simulink model "thermal_simulink_acados"  (R2017b)
settings: Solver=FixedStepDiscrete  StartTime=0.0  StopTime=500  FixedStep=1  RelTol=1e-3
values from neighbouring files (symbols this model uses):
  A_d = [0.386994154142 0.130528867937 0.00753731445977 1.05252849992e-06 0 0 0 0 0 0 0 -0.260915565234 ... (121 elements, 11x11)]    [battery_final_discrete_for_simulink.mat]    (also in convert_c2d.m = battery_sys_d.A)
  B_d = [0.00407902712304 0.000471082153736 1.68404559988e-05 1.71473651939e-09 0 0 0 0 0 0 0 0 ... (44 elements, 11x4)]    [battery_final_discrete_for_simulink.mat]    (also in convert_c2d.m = battery_sys_d.B)
  C_d = [-0.0403469184323 0 0.00489964923997 0 -0.00193385654799 0 0.0091411610057 0 0.0963442624262 0 0.00960199809146 0 ... (22 elements, 2x11)]    [battery_final_discrete_for_simulink.mat]    (also in convert_c2d.m = battery_sys_d.C)
  D_d = [0  0  0  0; 0  0  0  0]    [battery_final_discrete_for_simulink.mat]    (also in convert_c2d.m = battery_sys_d.D)
  nx_final = 11    [battery_final_portable_mux_demux_model.mat]
undefined symbols (not defined in the file or in its folder): DiscIntNeverNeededParam, disturbance_values
libraries: cstblocks x1, simulink x1
settings Model: Creator=dhruvkumar.patel  LastModifiedBy=dhruvkumar.patel

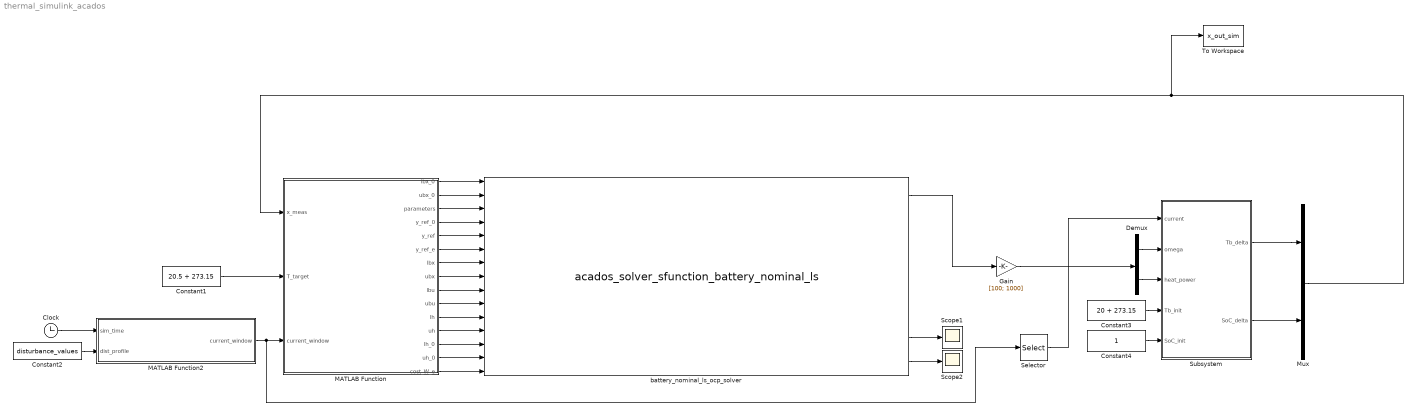
== system thermal_simulink_acados ==
  Clock : Clock
  Constant1 : Constant  Value=20.5 + 273.15
  Constant2 : Constant  Value=disturbance_values
  Constant3 : Constant  Value=20 + 273.15
  Constant4 : Constant
  Demux : Demux  Outputs=2
  Gain : Gain  Gain=[100; 1000]
  MATLAB Function : MATLAB Function  TreatAsAtomicUnit=on
  MATLAB Function2 : MATLAB Function  TreatAsAtomicUnit=on
  Mux : Mux  Inputs=2
  Scope1 : Scope
  Scope2 : Scope
  Selector : Selector  InputPortWidth=81  IndexOptions=Index vector (dialog)  Indices=1  OutputSizes=1
  Subsystem : Subsystem
  To Workspace : ToWorkspace  VariableName=x_out_sim  SampleTime=-1
  battery_nominal_ls_ocp_solver : S-Function  FunctionName=acados_solver_sfunction_battery_nominal_ls  SFunctionDeploymentMode=off  EnableBusSupport=off
      mask Display:
      | global sfun_input_names sfun_output_names
      | for i = 1:length(sfun_input_names)
      |     port_label('input', i, sfun_input_names{i})
      | end
      | for i = 1:length(sfun_output_names)
      |     port_label('output', i, sfun_output_names{i})
      | end
      | disp("acados OCP")
  wires:
  MATLAB Function/6(y_ref_e) -> battery_nominal_ls_ocp_solver/6
  MATLAB Function/5(y_ref) -> battery_nominal_ls_ocp_solver/5
  MATLAB Function/4(y_ref_0) -> battery_nominal_ls_ocp_solver/4
  MATLAB Function/3(parameters) -> battery_nominal_ls_ocp_solver/3
  MATLAB Function/2(ubx_0) -> battery_nominal_ls_ocp_solver/2
  MATLAB Function/1(lbx_0) -> battery_nominal_ls_ocp_solver/1
  MATLAB Function/7(lbx) -> battery_nominal_ls_ocp_solver/7
  MATLAB Function/8(ubx) -> battery_nominal_ls_ocp_solver/8
  MATLAB Function/9(lbu) -> battery_nominal_ls_ocp_solver/9
  MATLAB Function/10(ubu) -> battery_nominal_ls_ocp_solver/10
  MATLAB Function/11(lh) -> battery_nominal_ls_ocp_solver/11
  MATLAB Function/12(uh) -> battery_nominal_ls_ocp_solver/12
  MATLAB Function/13(lh_0) -> battery_nominal_ls_ocp_solver/13
  MATLAB Function/14(uh_0) -> battery_nominal_ls_ocp_solver/14
  MATLAB Function/15(cost_W_e) -> battery_nominal_ls_ocp_solver/15
  Constant1/1 -> MATLAB Function/2(T_target)
  MATLAB Function2/1(current_window) -> Selector/1, MATLAB Function/3(current_window)
  Clock/1 -> MATLAB Function2/1(sim_time)
  Constant2/1 -> MATLAB Function2/2(dist_profile)
  battery_nominal_ls_ocp_solver/7 -> Scope1/1
  battery_nominal_ls_ocp_solver/8 -> Scope2/1
  battery_nominal_ls_ocp_solver/1 -> Gain/1
  Gain/1 -> Demux/1
  Demux/1 -> Subsystem/2(omega)
  Demux/2 -> Subsystem/3(heat_power)
  Selector/1 -> Subsystem/1(current)
  Mux/1 -> To Workspace/1, MATLAB Function/1(x_meas)
  Subsystem/1(Tb_delta) -> Mux/1
  Subsystem/2(SoC_delta) -> Mux/2
  Constant3/1 -> Subsystem/4(Tb_init)
  Constant4/1 -> Subsystem/5(SoC_init)

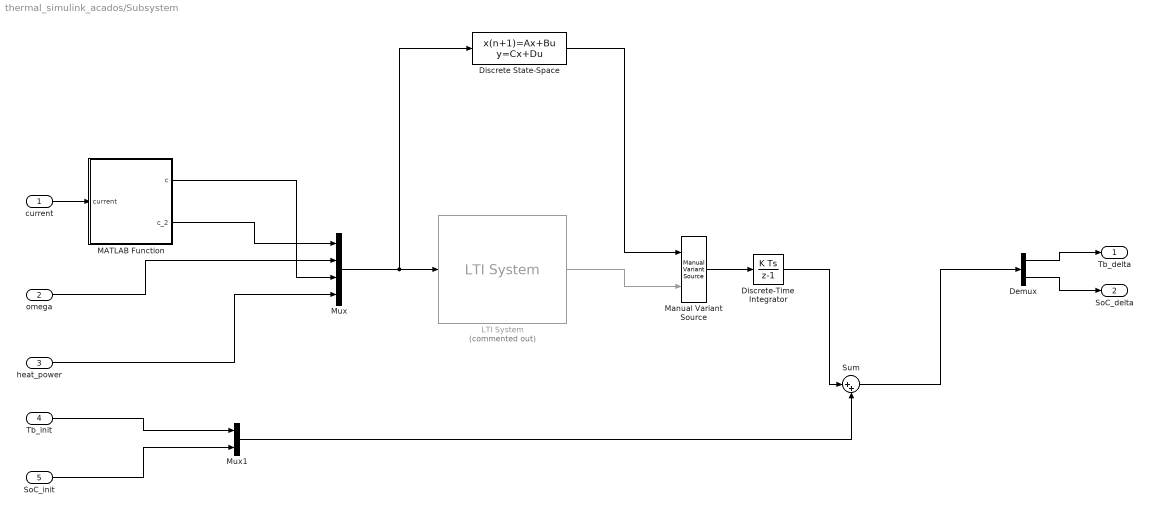
== system thermal_simulink_acados/Subsystem ==
  current : Inport
  omega : Inport  Port=2
  heat_power : Inport  Port=3
  Tb_init : Inport  Port=4
  SoC_init : Inport  Port=5
  Demux : Demux  Outputs=2
  Discrete State-Space : DiscreteStateSpace  A=A_d  B=B_d  C=C_d  D=D_d  InitialCondition=zeros(nx_final,1)  SampleTime=-1
  Discrete-Time Integrator : DiscreteIntegrator  InitialConditionSetting=State (most efficient)  SampleTime=-1  ICPrevOutput=DiscIntNeverNeededParam  ICPrevScaledInput=DiscIntNeverNeededParam
  LTI System : cstblocks/LTI System  Commented=on  sys=TF_final  IC=[]
  MATLAB Function : MATLAB Function  TreatAsAtomicUnit=on
  Manual Variant Source : simulink/Signal Routing/Manual Variant Source  NumChoices=2  OverrideUsingVariant=V_1
      settings: SourceProductName=Simulink
  Mux : Mux
  Mux1 : Mux  Inputs=2
  Sum : Sum  Inputs=|++
  Tb_delta : Outport
  SoC_delta : Outport  Port=2
  wires:
  current/1 -> MATLAB Function/1(current)
  Mux/1 -> Discrete State-Space/1, LTI System/1
  MATLAB Function/1(c) -> Mux/3
  Demux/2 -> SoC_delta/1
  Demux/1 -> Tb_delta/1
  MATLAB Function/2(c_2) -> Mux/1
  Manual Variant Source/1 -> Discrete-Time Integrator/1
  heat_power/1 -> Mux/4
  omega/1 -> Mux/2
  Discrete State-Space/1 -> Manual Variant Source/1
  LTI System/1 -> Manual Variant Source/2
  Tb_init/1 -> Mux1/1
  SoC_init/1 -> Mux1/2
  Discrete-Time Integrator/1 -> Sum/1
  Mux1/1 -> Sum/2
  Sum/1 -> Demux/1

== matlab function thermal_simulink_acados/Subsystem/MATLAB Function ==
  data: current input; c output; c_2 output
function [c,c_2] = fcn(current)
c_2=current^2;
c=current;
end

== matlab function thermal_simulink_acados/MATLAB Function ==
  data: x_meas input; lbx_0 output; T_target input; current_window input; ubx_0 output; parameters output; y_ref_0 output; y_ref output; y_ref_e output; lbx output; ubx output; lbu output; ubu output; lh output; uh output; lh_0 output; uh_0 output; cost_W_e output
function [lbx_0, ubx_0, parameters, y_ref_0, y_ref, y_ref_e, lbx, ubx, lbu, ubu, lh, uh, lh_0, uh_0, cost_W_e] = prep_acados_inputs(x_meas, T_target, current_window)
    % Inputs:
    % x_meas: Current battery state [T_bat; SOC] (Size: 2x1)
    % T_target: Target temperature in Kelvin (Size: 1x1)
    % current_window: Disturbance forecast for the horizon (Size: 81x1)
    CELSIUS_TO_KELVIN = 273.15;
    
    %% 1. Initial State Constraint (lbx_0 and ubx_0)
    % By setting both lower and upper bounds to the measured state, 
    % we force the solver to start exactly at the current physical state.
    lbx_0 = x_meas;
    ubx_0 = x_meas;
    
    %% 2. References
    omega_ss = 0.5;  % Steady state pump
    Q_heat_ss = 0.0; % Steady state heater
    
    % Stage 0 (Size: 4)
    % Notice we use x_meas(2) for SOC reference so the error is always 0
    y_ref_0 = [T_target; x_meas(2); omega_ss; Q_heat_ss];
    
    % Stages 1 to N-1 (Size: 316 = 79 * 4)
    y_ref_step = [T_target; x_meas(2); omega_ss; Q_heat_ss];
    y_ref = repmat(y_ref_step, 79, 1); % Duplicate the step 79 times
    
    % Terminal Stage (Size: 2)
    y_ref_e = [T_target; x_meas(2)];
    
    %% 3. Parameters
    % The disturbance parameter passed directly (Size: 81)
    parameters = current_window; 

    %% 4. State Bounds (Stages 1 to N-1, Size: 79)
    % Note: Only T_bat is constrained in your Python setup, but check if your 
    % Simulink block expects both states. Assuming only T_bat here:
    Tb_min = -20 + CELSIUS_TO_KELVIN;
    Tb_max = 50 + CELSIUS_TO_KELVIN;
    lbx = repmat(Tb_min, 79, 1);
    ubx = repmat(Tb_max, 79, 1);
    
    %% 5. Control Bounds (Stages 0 to N-1, Size: 160 = 80 * 2)
    omega_min = (150*2*pi/60)/100;   omega_max = (4000*2*pi/60)/100;
    Q_heat_min = -4000/1000;         Q_heat_max = 4000/1000;
    
    u_min_step = [omega_min; Q_heat_min];
    u_max_step = [omega_max; Q_heat_max];
    lbu = repmat(u_min_step, 80, 1);
    ubu = repmat(u_max_step, 80, 1);
    
    %% 6. Nonlinear Bounds (T_clin, T_clout)
    h_min = [-20 + CELSIUS_TO_KELVIN; -20 + CELSIUS_TO_KELVIN];
    h_max = [100 + CELSIUS_TO_KELVIN; 100 + CELSIUS_TO_KELVIN];
    
    %% 7. Stages 1 to N-1 (Size: 158 = 79 * 2)
    lh = repmat(h_min, 79, 1);
    uh = repmat(h_max, 79, 1);
    
    %% 8. Stage 0 (Size: 2)
    lh_0 = h_min;
    uh_0 = h_max;

    %% Tterminal cost matrix
    % P_lqr_matrix is passed in, and we append the SOC weight (e.g., 0.1)
    Q_e = [859.3722, 0; 
           0,            0.1];
           
    % Flatten to column-major [4x1] for the Acados S-Function
    cost_W_e = Q_e(:);
end

== matlab function thermal_simulink_acados/MATLAB Function2 ==
  data: sim_time input; current_window output; dist_profile input
function current_window = get_disturbance_window(sim_time, dist_profile)
    % dist_profile is now passed as an input/parameter directly from Simulink!
    
    % Assuming a 1-second sample time
    current_idx = floor(sim_time) + 1; 
    
    % Extract current step + 80 future steps (Size: 81x1)
    current_window = dist_profile(current_idx : current_idx + 80);
end
